simulink model "untitled"  (Simulink 10.3)
settings: Solver=ode45  StartTime=0.0  StopTime=10.0  RelTol=1e-3  EnableMultiTasking=on
libraries: dsparch4 x3, dspstat3 x1, dspmathops x1
settings Model: Creator=27734  LastModifiedBy=27734
settings SolverCC: AlgebraicLoopSolver=Auto
settings DataIOCC: LimitDataPoints=on  SignalLoggingName=sigsOut
settings OptimizationCC: ExpressionDepthLimit=128  LifeSpan=auto
settings DebuggingCC: SaveWithParameterizedLinksMsg=none  SignalResolutionControl=TryResolveAllWithWarning  MultiTaskDSMMsg=warning  MultiTaskCondExecSysMsg=none  FcnCallInpInsideContextMsg=error  StateNameClashWarn=none  SFUnexpectedBacktrackingDiag=error  SFNoUnconditionalDefaultTransitionDiag=error  SFExecutionAtInitializationDiag=warning  SFMachineParentedDataDiag=error  ArithmeticOperatorsInVariantConditions=error
settings HardwareCC: TargetUnknown=on
settings SFSimCC: SimUseLocalCustomCode=on  CustomCodeUndefinedFunction=FilterOut
settings RTWCC: RTWUseLocalCustomCode=on
settings CodeAppCC: StateflowObjectComments=off
settings GRTTargetCC: TargetLangStandard=C99 (ISO)
settings ConfigComp: CovExternalEMLEnable=on

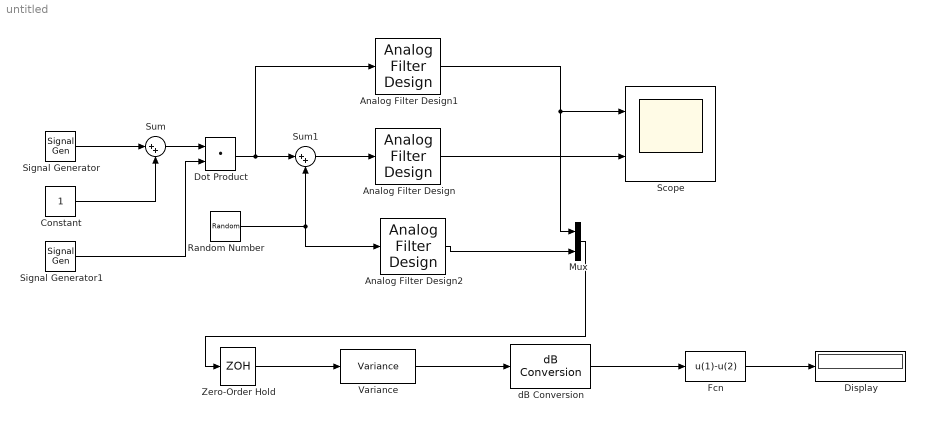
== system untitled ==
  Analog Filter Design : dsparch4/Analog Filter Design  method=Butterworth  filttype=Bandpass  N=2  Wlo=2*pi*(1e6-6e3)  Whi=2*pi*(1e6+6e3)  Rp=2  Rs=40
  Analog Filter Design1 : dsparch4/Analog Filter Design  method=Butterworth  filttype=Bandpass  N=2  Wlo=2*pi*(1e6-6e3)  Whi=2*pi*(1e6+6e3)  Rp=2  Rs=40
  Analog Filter Design2 : dsparch4/Analog Filter Design  method=Butterworth  filttype=Bandpass  N=2  Wlo=2*pi*(1e6-6e3)  Whi=2*pi*(1e6+6e3)  Rp=2  Rs=40
  Constant : Constant
  Display : Display
  Dot Product : DotProduct  InputSameDT=on  OutDataTypeStr=Inherit: Inherit via internal rule
  Fcn : Fcn  Expr=u(1)-u(2)
  Mux : Mux  Inputs=2
  Random Number : RandomNumber  Variance=3.4945  SampleTime=6.23e-8
  Scope : Scope  NumInputPorts=2
  Signal Generator : SignalGenerator  Amplitude=0.3  Frequency=1000
  Signal Generator1 : SignalGenerator  Frequency=1000000
  Sum : Sum  Inputs=|++  SaturateOnIntegerOverflow=on
  Sum1 : Sum  Inputs=|++  SaturateOnIntegerOverflow=on
  Variance : dspstat3/Variance  run=on  InputProcessing=Columns as channels (frame based)  reset_popup=None  directionMode=Each column  dimension=1  roiEnable=off  roiType=Rectangles  roiPortion=Entire ROI  roiOutput=Individual statistics for each ROI  roiFlag=off  roundingMode=Floor  overflowMode=off
  Zero-Order Hold : ZeroOrderHold  SampleTime=6.23e-8
  dB Conversion : dspmathops/dB Conversion  dBtype=dB  intype=Power  R=1  fuzz=on
  wires:
  Signal Generator/1 -> Sum/1
  Constant/1 -> Sum/2
  Sum/1 -> Dot Product/1
  Signal Generator1/1 -> Dot Product/2
  Dot Product/1 -> Analog Filter Design1/1, Sum1/1
  Sum1/1 -> Analog Filter Design/1
  dB Conversion/1 -> Fcn/1
  Fcn/1 -> Display/1
  Analog Filter Design2/1 -> Mux/2
  Analog Filter Design1/1 -> Mux/1, Scope/1
  Mux/1 -> Zero-Order Hold/1
  Analog Filter Design/1 -> Scope/2
  Zero-Order Hold/1 -> Variance/1
  Variance/1 -> dB Conversion/1
  Random Number/1 -> Analog Filter Design2/1, Sum1/2
